simulink model "p1_digital_twin_R2023a"  (R2023a)
settings: Solver=FixedStepDiscrete  StartTime=0.0  StopTime=10  FixedStep=Ts  RelTol=1e-3  EnableMultiTasking=on
values from neighbouring files (symbols this model uses):
  ack = 1    [SteeringController.m]
  cpr_handwheel = 500*4    (= 2000)    [p1_params_new.m]
  cpr_steering = 1000*4    (= 4000)    [p1_params_new.m]
  hal_filter_den = [1 1*(2*pi*Ts)-1]    [SteeringController.m]    (also in p1_params_new.m = DEN_cellarray{1})
  hal_filter_num = [1*(2*pi*Ts)]    [SteeringController.m]    (also in p1_params_new.m = NUM_cellarray{1})
  n_drive = 5.6    [p1_params_new.m]
  n_handwheel = 50    [p1_params_new.m]
  n_steering = 160    [p1_params_new.m]
  sr = 7.5    [SteeringController.m]
  steering_limit = 35    [SteeringController.m]
  Ts = 0.001    [p1_params_new.m]
  wc = 10    [SteeringController.m]    (also in p1_params_new.m = p1params.input.VAccelFc*(2*Ts))
undefined symbols (not defined in the file or in its folder): DiscIntNeverNeededParam, p1params, param
libraries: simulink x7
(part 3 of 4)

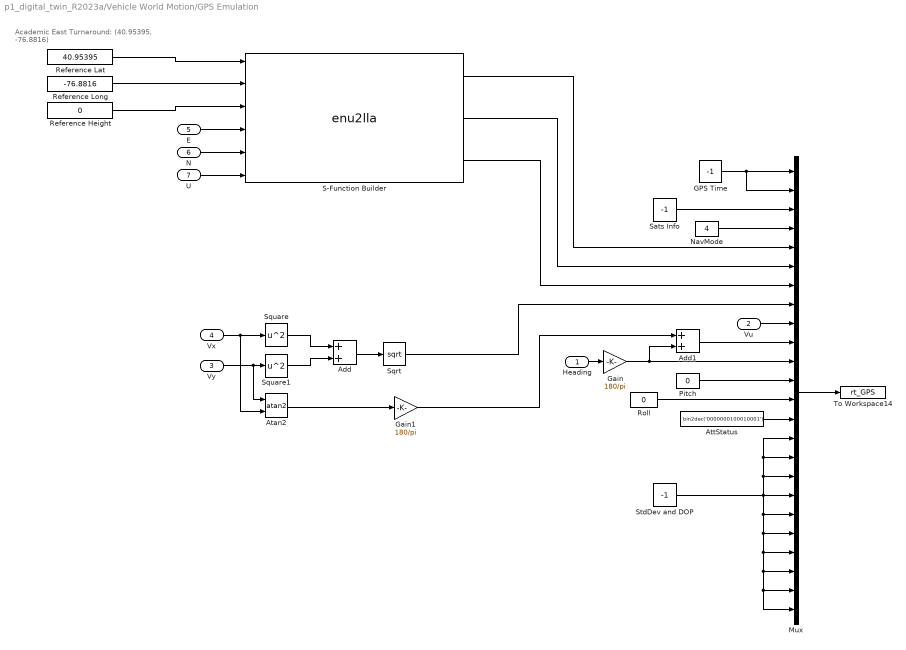
== system p1_digital_twin_R2023a/Vehicle World Motion/GPS Emulation ==
  note: Academic East Turnaround:
      | (40.95395, -76.8816)
  Heading : Inport
  Vu : Inport  Port=2
  Vy : Inport  Port=3
  Vx : Inport  Port=4
  E : Inport  Port=5
  N : Inport  Port=6
  U : Inport  Port=7
  Add : Sum
  Add1 : Sum
  Atan2 : Trigonometry  Operator=atan2
  AttStatus : Constant  Value=bin2dec('0000000100010001')  OutDataTypeStr=double
  GPS Time : Constant  Value=-1
  Gain : Gain  Gain=180/pi
  Gain1 : Gain  Gain=180/pi
  Mux : Mux  Inputs=24
  NavMode : Constant  Value=4
  Pitch : Constant  Value=0
  Reference Height : Constant  Value=0
  Reference Lat : Constant  Value=40.95395
  Reference Long : Constant  Value=-76.8816
  Roll : Constant  Value=0
  S-Function Builder : S-Function  FunctionName=enu2lla  SFunctionModules=enu2lla_wrapper.c  SFunctionDeploymentMode=off  EnableBusSupport=off  mask(S-Function Builder){}
      mask help: Simulink:masks:SFunctionBuilder_MD
      mask init: same as p1_digital_twin_R2023a/Actuator Dynamics/Steering System Emulation/S-Function Builder1
      settings: CopyFcn=set_param(gcbh,'LinkStatus','none')  OpenFcn=sfunctionwizard(gcbh)
      mask Display:
      | plot(val(:,1),val(:,2))
      | disp(sys)
      | port_label('input',1,'u0')
      | port_label('input',2,'u1')
      | port_label('input',3,'u2')
      | port_label('input',4,'u3')
      | port_label('input',5,'u4')
      | port_label('input',6,'u5')
      | port_label('output',1,'y0')
      | port_label('output',2,'y1')
      | port_label('output',3,'y2')
  Sats Info : Constant  Value=-1
  Sqrt : Sqrt
  Square : Math  Operator=square
  Square1 : Math  Operator=square
  StdDev and DOP : Constant  Value=-1
  To Workspace14 : ToWorkspace  VariableName=rt_GPS  SampleTime=-1
  wires:
  Add/1 -> Sqrt/1
  Vy/1 -> Atan2/1, Square1/1
  Vx/1 -> Atan2/2, Square/1
  Square/1 -> Add/1
  Square1/1 -> Add/2
  GPS Time/1 -> Mux/1, Mux/2
  NavMode/1 -> Mux/4
  S-Function Builder/1 -> Mux/5
  Sqrt/1 -> Mux/8
  Vu/1 -> Mux/9
  S-Function Builder/2 -> Mux/6
  S-Function Builder/3 -> Mux/7
  Pitch/1 -> Mux/12
  AttStatus/1 -> Mux/14
  Heading/1 -> Gain/1
  StdDev and DOP/1 -> Mux/18, Mux/17, Mux/16, Mux/15, Mux/19, Mux/20, Mux/21, Mux/22, Mux/23, Mux/24
  Sats Info/1 -> Mux/3
  Mux/1 -> To Workspace14/1
  Roll/1 -> Mux/13
  Gain/1 -> Add1/2, Mux/11
  Atan2/1 -> Gain1/1
  Add1/1 -> Mux/10
  Gain1/1 -> Add1/1
  Reference Lat/1 -> S-Function Builder/1
  Reference Long/1 -> S-Function Builder/2
  Reference Height/1 -> S-Function Builder/3
  E/1 -> S-Function Builder/4
  U/1 -> S-Function Builder/6
  N/1 -> S-Function Builder/5

== system p1_digital_twin_R2023a/Vehicle World Motion/IMU Emulation1 ==
  note: Filtering Operations from IMU?
  note: Break into bytes
  Roll Rate : Inport
  Pitch Rate : Inport  Port=2
  Yaw Rate : Inport  Port=3
  Ax : Inport  Port=4
  Ay : Inport  Port=5
  Az : Inport  Port=6
  Accel unscaling : Gain  Gain=32768/(2*9.81)
  Accel unscaling1 : Gain  Gain=32768/(2*9.81)
  Accel unscaling2 : Gain  Gain=32768/(2*9.81)
  Data Type Conversion{,1..5} (6 alike) : DataTypeConversion  OutDataTypeStr=int16  SaturateOnIntegerOverflow=off  RndMeth=Floor
  Gyro unscaling : Gain  Gain=32768/(500*pi/180)
  Gyro unscaling1 : Gain  Gain=32768/500
  Gyro unscaling2 : Gain  Gain=32768/500
  Mux : Mux  Inputs=12
  S-Function Builder : S-Function  FunctionName=int16ToBytes  SFunctionModules=int16ToBytes_wrapper.c  SFunctionDeploymentMode=off  EnableBusSupport=off  mask(S-Function Builder){}
      mask help: Simulink:masks:SFunctionBuilder_MD
      mask init: same as p1_digital_twin_R2023a/Actuator Dynamics/Steering System Emulation/S-Function Builder1
      settings: CopyFcn=set_param(gcbh,'LinkStatus','none')  OpenFcn=sfunctionwizard(gcbh)
      mask Display:
      | plot(val(:,1),val(:,2))
      | disp(sys)
      | port_label('input',1,'u0')
      | port_label('output',1,'y0')
  S-Function Builder1 : S-Function  FunctionName=int16ToBytes  SFunctionModules=int16ToBytes_wrapper.c  SFunctionDeploymentMode=off  EnableBusSupport=off  mask(S-Function Builder){}
      mask help: Simulink:masks:SFunctionBuilder_MD
      mask init: same as p1_digital_twin_R2023a/Actuator Dynamics/Steering System Emulation/S-Function Builder1
      settings: CopyFcn=set_param(gcbh,'LinkStatus','none')  OpenFcn=sfunctionwizard(gcbh)
      mask Display:
      | plot(val(:,1),val(:,2))
      | disp(sys)
      | port_label('input',1,'u0')
      | port_label('output',1,'y0')
  S-Function Builder2 : S-Function  FunctionName=int16ToBytes  SFunctionModules=int16ToBytes_wrapper.c  SFunctionDeploymentMode=off  EnableBusSupport=off  mask(S-Function Builder){}
      mask help: Simulink:masks:SFunctionBuilder_MD
      mask init: same as p1_digital_twin_R2023a/Actuator Dynamics/Steering System Emulation/S-Function Builder1
      settings: CopyFcn=set_param(gcbh,'LinkStatus','none')  OpenFcn=sfunctionwizard(gcbh)
      mask Display:
      | plot(val(:,1),val(:,2))
      | disp(sys)
      | port_label('input',1,'u0')
      | port_label('output',1,'y0')
      | port_label('output',2,'y1')
  S-Function Builder3 : S-Function  FunctionName=int16ToBytes  SFunctionModules=int16ToBytes_wrapper.c  SFunctionDeploymentMode=off  EnableBusSupport=off  mask(S-Function Builder){}
      mask help: Simulink:masks:SFunctionBuilder_MD
      mask init: same as p1_digital_twin_R2023a/Actuator Dynamics/Steering System Emulation/S-Function Builder1
      settings: CopyFcn=set_param(gcbh,'LinkStatus','none')  OpenFcn=sfunctionwizard(gcbh)
      mask Display:
      | plot(val(:,1),val(:,2))
      | disp(sys)
      | port_label('input',1,'u0')
      | port_label('output',1,'y0')
  S-Function Builder4 : S-Function  FunctionName=int16ToBytes  SFunctionModules=int16ToBytes_wrapper.c  SFunctionDeploymentMode=off  EnableBusSupport=off  mask(S-Function Builder){}
      mask help: Simulink:masks:SFunctionBuilder_MD
      mask init: same as p1_digital_twin_R2023a/Actuator Dynamics/Steering System Emulation/S-Function Builder1
      settings: CopyFcn=set_param(gcbh,'LinkStatus','none')  OpenFcn=sfunctionwizard(gcbh)
      mask Display:
      | plot(val(:,1),val(:,2))
      | disp(sys)
      | port_label('input',1,'u0')
      | port_label('output',1,'y0')
  S-Function Builder5 : S-Function  FunctionName=int16ToBytes  SFunctionModules=int16ToBytes_wrapper.c  SFunctionDeploymentMode=off  EnableBusSupport=off  mask(S-Function Builder){}
      mask help: Simulink:masks:SFunctionBuilder_MD
      mask init: same as p1_digital_twin_R2023a/Actuator Dynamics/Steering System Emulation/S-Function Builder1
      settings: CopyFcn=set_param(gcbh,'LinkStatus','none')  OpenFcn=sfunctionwizard(gcbh)
      mask Display:
      | plot(val(:,1),val(:,2))
      | disp(sys)
      | port_label('input',1,'u0')
      | port_label('output',1,'y0')
  To Workspace16 : ToWorkspace  VariableName=rt_IMU  SampleTime=-1
      settings: Save2DSignal=2-D array (concatenate along first dimension)
  wires:
  Mux/1 -> To Workspace16/1
  Accel unscaling/1 -> Data Type Conversion3/1
  Accel unscaling1/1 -> Data Type Conversion4/1
  Accel unscaling2/1 -> Data Type Conversion5/1
  Gyro unscaling2/1 -> Data Type Conversion2/1
  Pitch Rate/1 -> Gyro unscaling1/1
  Yaw Rate/1 -> Gyro unscaling/1
  Gyro unscaling1/1 -> Data Type Conversion1/1
  Gyro unscaling/1 -> Data Type Conversion/1
  Roll Rate/1 -> Gyro unscaling2/1
  Az/1 -> Accel unscaling2/1
  Ay/1 -> Accel unscaling1/1
  Ax/1 -> Accel unscaling/1
  Data Type Conversion/1 -> S-Function Builder/1
  Data Type Conversion2/1 -> S-Function Builder2/1
  Data Type Conversion1/1 -> S-Function Builder1/1
  Data Type Conversion3/1 -> S-Function Builder3/1
  Data Type Conversion4/1 -> S-Function Builder4/1
  Data Type Conversion5/1 -> S-Function Builder5/1
  S-Function Builder5/1 -> Mux/11, Mux/12
  S-Function Builder2/1 -> Mux/1, Mux/2
  S-Function Builder1/1 -> Mux/3, Mux/4
  S-Function Builder/1 -> Mux/5, Mux/6
  S-Function Builder3/1 -> Mux/7, Mux/8
  S-Function Builder4/1 -> Mux/9, Mux/10

== system p1_digital_twin_R2023a/Actuator Dynamics/Drivetrain Emulation/Accurate Feedback L ==
  Actual Torque : Inport
  Actual Voltage : Inport  Port=2
  Actual Current : Inport  Port=3
  Actual Speed : Inport  Port=4
  Bias1 : Bias  Bias=3212.8  SaturateOnIntegerOverflow=off
  Bias2 : Bias  Bias=3212.8  SaturateOnIntegerOverflow=off
  Bias3 : Bias  Bias=16064  SaturateOnIntegerOverflow=off
  Data Type Conversion{1..3,5} (4 alike) : DataTypeConversion  OutDataTypeStr=uint16  SaturateOnIntegerOverflow=off  RndMeth=Floor
  Mux{,1,3..4} (4 alike) : Mux  Inputs=2
  Mux2 : Mux
  S-Function Builder : S-Function  FunctionName=uint16ToBytes  SFunctionModules=uint16ToBytes_wrapper.c  SFunctionDeploymentMode=off  EnableBusSupport=off  mask(S-Function Builder){}
      mask help: Simulink:masks:SFunctionBuilder_MD
      mask init: same as p1_digital_twin_R2023a/Actuator Dynamics/Steering System Emulation/S-Function Builder1
      settings: CopyFcn=set_param(gcbh,'LinkStatus','none')  OpenFcn=sfunctionwizard(gcbh)
      mask Display:
      | plot(val(:,1),val(:,2))
      | disp(sys)
      | port_label('input',1,'u0')
      | port_label('output',1,'y0')
      | port_label('output',2,'y1')
  S-Function Builder1 : S-Function  FunctionName=uint16ToBytes  SFunctionModules=uint16ToBytes_wrapper.c  SFunctionDeploymentMode=off  EnableBusSupport=off  mask(S-Function Builder){}
      mask help: Simulink:masks:SFunctionBuilder_MD
      mask init: same as p1_digital_twin_R2023a/Actuator Dynamics/Steering System Emulation/S-Function Builder1
      settings: CopyFcn=set_param(gcbh,'LinkStatus','none')  OpenFcn=sfunctionwizard(gcbh)
      mask Display:
      | plot(val(:,1),val(:,2))
      | disp(sys)
      | port_label('input',1,'u0')
      | port_label('output',1,'y0')
      | port_label('output',2,'y1')
  S-Function Builder2 : S-Function  FunctionName=uint16ToBytes  SFunctionModules=uint16ToBytes_wrapper.c  SFunctionDeploymentMode=off  EnableBusSupport=off  mask(S-Function Builder){}
      mask help: Simulink:masks:SFunctionBuilder_MD
      mask init: same as p1_digital_twin_R2023a/Actuator Dynamics/Steering System Emulation/S-Function Builder1
      settings: CopyFcn=set_param(gcbh,'LinkStatus','none')  OpenFcn=sfunctionwizard(gcbh)
      mask Display:
      | plot(val(:,1),val(:,2))
      | disp(sys)
      | port_label('input',1,'u0')
      | port_label('output',1,'y0')
      | port_label('output',2,'y1')
  S-Function Builder3 : S-Function  FunctionName=uint16ToBytes  SFunctionModules=uint16ToBytes_wrapper.c  SFunctionDeploymentMode=off  EnableBusSupport=off  mask(S-Function Builder){}
      mask help: Simulink:masks:SFunctionBuilder_MD
      mask init: same as p1_digital_twin_R2023a/Actuator Dynamics/Steering System Emulation/S-Function Builder1
      settings: CopyFcn=set_param(gcbh,'LinkStatus','none')  OpenFcn=sfunctionwizard(gcbh)
      mask Display:
      | plot(val(:,1),val(:,2))
      | disp(sys)
      | port_label('input',1,'u0')
      | port_label('output',1,'y0')
      | port_label('output',2,'y1')
  Speed scaling1 : Gain  Gain=1/.1
  Speed scaling2 : Gain  Gain=1/.1
  Speed scaling3 : Gain  Gain=1/.5
  Torque offset : Bias  Bias=+3212.8  SaturateOnIntegerOverflow=off
  Torque scaling : Gain  Gain=1/.1
  Out2 : Outport
  wires:
  Mux2/1 -> Out2/1
  Actual Torque/1 -> Torque offset/1
  Torque scaling/1 -> Data Type Conversion5/1
  Data Type Conversion5/1 -> S-Function Builder3/1
  S-Function Builder3/2 -> Mux/2
  S-Function Builder3/1 -> Mux/1
  Mux/1 -> Mux2/1
  S-Function Builder2/1 -> Mux1/1
  Speed scaling1/1 -> Data Type Conversion1/1
  Actual Voltage/1 -> Bias1/1
  S-Function Builder2/2 -> Mux1/2
  Mux1/1 -> Mux2/2
  Data Type Conversion1/1 -> S-Function Builder2/1
  S-Function Builder1/2 -> Mux3/2
  Speed scaling2/1 -> Data Type Conversion2/1
  Data Type Conversion2/1 -> S-Function Builder1/1
  Actual Current/1 -> Bias2/1
  S-Function Builder1/1 -> Mux3/1
  Mux3/1 -> Mux2/3
  Torque offset/1 -> Torque scaling/1
  Bias1/1 -> Speed scaling1/1
  Bias2/1 -> Speed scaling2/1
  S-Function Builder/2 -> Mux4/2
  Mux4/1 -> Mux2/4
  Speed scaling3/1 -> Data Type Conversion3/1
  Data Type Conversion3/1 -> S-Function Builder/1
  Bias3/1 -> Speed scaling3/1
  Actual Speed/1 -> Bias3/1
  S-Function Builder/1 -> Mux4/1

== system p1_digital_twin_R2023a/Actuator Dynamics/Drivetrain Emulation/Accurate Feedback R ==
  Actual Torque : Inport
  Actual Voltage : Inport  Port=2
  Actual Current : Inport  Port=3
  Actual Speed : Inport  Port=4
  Bias1 : Bias  Bias=3212.8  SaturateOnIntegerOverflow=off
  Bias2 : Bias  Bias=3212.8  SaturateOnIntegerOverflow=off
  Bias3 : Bias  Bias=16064  SaturateOnIntegerOverflow=off
  Data Type Conversion{1..3,5} (4 alike) : DataTypeConversion  OutDataTypeStr=uint16  SaturateOnIntegerOverflow=off  RndMeth=Floor
  Mux{,1,3..4} (4 alike) : Mux  Inputs=2
  Mux2 : Mux
  S-Function Builder : S-Function  FunctionName=uint16ToBytes  SFunctionModules=uint16ToBytes_wrapper.c  SFunctionDeploymentMode=off  EnableBusSupport=off  mask(S-Function Builder){}
      mask help: Simulink:masks:SFunctionBuilder_MD
      mask init: same as p1_digital_twin_R2023a/Actuator Dynamics/Steering System Emulation/S-Function Builder1
      settings: CopyFcn=set_param(gcbh,'LinkStatus','none')  OpenFcn=sfunctionwizard(gcbh)
      mask Display:
      | plot(val(:,1),val(:,2))
      | disp(sys)
      | port_label('input',1,'u0')
      | port_label('output',1,'y0')
      | port_label('output',2,'y1')
  S-Function Builder1 : S-Function  FunctionName=uint16ToBytes  SFunctionModules=uint16ToBytes_wrapper.c  SFunctionDeploymentMode=off  EnableBusSupport=off  mask(S-Function Builder){}
      mask help: Simulink:masks:SFunctionBuilder_MD
      mask init: same as p1_digital_twin_R2023a/Actuator Dynamics/Steering System Emulation/S-Function Builder1
      settings: CopyFcn=set_param(gcbh,'LinkStatus','none')  OpenFcn=sfunctionwizard(gcbh)
      mask Display:
      | plot(val(:,1),val(:,2))
      | disp(sys)
      | port_label('input',1,'u0')
      | port_label('output',1,'y0')
      | port_label('output',2,'y1')
  S-Function Builder2 : S-Function  FunctionName=uint16ToBytes  SFunctionModules=uint16ToBytes_wrapper.c  SFunctionDeploymentMode=off  EnableBusSupport=off  mask(S-Function Builder){}
      mask help: Simulink:masks:SFunctionBuilder_MD
      mask init: same as p1_digital_twin_R2023a/Actuator Dynamics/Steering System Emulation/S-Function Builder1
      settings: CopyFcn=set_param(gcbh,'LinkStatus','none')  OpenFcn=sfunctionwizard(gcbh)
      mask Display:
      | plot(val(:,1),val(:,2))
      | disp(sys)
      | port_label('input',1,'u0')
      | port_label('output',1,'y0')
      | port_label('output',2,'y1')
  S-Function Builder3 : S-Function  FunctionName=uint16ToBytes  SFunctionModules=uint16ToBytes_wrapper.c  SFunctionDeploymentMode=off  EnableBusSupport=off  mask(S-Function Builder){}
      mask help: Simulink:masks:SFunctionBuilder_MD
      mask init: same as p1_digital_twin_R2023a/Actuator Dynamics/Steering System Emulation/S-Function Builder1
      settings: CopyFcn=set_param(gcbh,'LinkStatus','none')  OpenFcn=sfunctionwizard(gcbh)
      mask Display:
      | plot(val(:,1),val(:,2))
      | disp(sys)
      | port_label('input',1,'u0')
      | port_label('output',1,'y0')
      | port_label('output',2,'y1')
  Speed scaling1 : Gain  Gain=1/.1
  Speed scaling2 : Gain  Gain=1/.1
  Speed scaling3 : Gain  Gain=1/.5
  Torque offset : Bias  Bias=+3212.8  SaturateOnIntegerOverflow=off
  Torque scaling : Gain  Gain=1/.1
  Out2 : Outport
  wires:
  Mux2/1 -> Out2/1
  Actual Torque/1 -> Torque offset/1
  Torque scaling/1 -> Data Type Conversion5/1
  Data Type Conversion5/1 -> S-Function Builder3/1
  S-Function Builder3/2 -> Mux/2
  S-Function Builder3/1 -> Mux/1
  Mux/1 -> Mux2/1
  S-Function Builder2/1 -> Mux1/1
  Speed scaling1/1 -> Data Type Conversion1/1
  Actual Voltage/1 -> Bias1/1
  S-Function Builder2/2 -> Mux1/2
  Mux1/1 -> Mux2/2
  Data Type Conversion1/1 -> S-Function Builder2/1
  S-Function Builder1/2 -> Mux3/2
  Speed scaling2/1 -> Data Type Conversion2/1
  Data Type Conversion2/1 -> S-Function Builder1/1
  Actual Current/1 -> Bias2/1
  S-Function Builder1/1 -> Mux3/1
  Mux3/1 -> Mux2/3
  Torque offset/1 -> Torque scaling/1
  Bias1/1 -> Speed scaling1/1
  Bias2/1 -> Speed scaling2/1
  S-Function Builder/2 -> Mux4/2
  Mux4/1 -> Mux2/4
  Speed scaling3/1 -> Data Type Conversion3/1
  Data Type Conversion3/1 -> S-Function Builder/1
  Bias3/1 -> Speed scaling3/1
  Actual Speed/1 -> Bias3/1
  S-Function Builder/1 -> Mux4/1

== system p1_digital_twin_R2023a/Actuator Dynamics/Drivetrain Emulation/Universal Command L ==
  Torque Request : Inport
  Fwd Speed Lim : Inport  Port=2
  Rev Speed Lim : Inport  Port=3
  Bias1 : Bias  Bias=16064  SaturateOnIntegerOverflow=off
  Bias2 : Bias  Bias=16064  SaturateOnIntegerOverflow=off
  Control Mode : Constant  Value=hex2dec('01')  OutDataTypeStr=uint8  SampleTime=-1
  Control Params : Constant  Value=bin2dec('00011000')  OutDataTypeStr=uint8  SampleTime=-1
  Data Type Conversion1 : DataTypeConversion  OutDataTypeStr=uint16  RndMeth=Floor
  Data Type Conversion2 : DataTypeConversion  OutDataTypeStr=uint16  SaturateOnIntegerOverflow=off  RndMeth=Floor
  Data Type Conversion5 : DataTypeConversion  OutDataTypeStr=uint16  SaturateOnIntegerOverflow=off  RndMeth=Floor
  Mux : Mux  Inputs=2
  Mux1 : Mux  Inputs=2
  Mux2 : Mux  Inputs=5
  Mux3 : Mux  Inputs=2
  S-Function Builder1 : S-Function  FunctionName=uint16ToBytes  SFunctionModules=uint16ToBytes_wrapper.c  SFunctionDeploymentMode=off  EnableBusSupport=off  mask(S-Function Builder){}
      mask help: Simulink:masks:SFunctionBuilder_MD
      mask init: same as p1_digital_twin_R2023a/Actuator Dynamics/Steering System Emulation/S-Function Builder1
      settings: CopyFcn=set_param(gcbh,'LinkStatus','none')  OpenFcn=sfunctionwizard(gcbh)
      mask Display:
      | plot(val(:,1),val(:,2))
      | disp(sys)
      | port_label('input',1,'u0')
      | port_label('output',1,'y0')
      | port_label('output',2,'y1')
  S-Function Builder2 : S-Function  FunctionName=uint16ToBytes  SFunctionModules=uint16ToBytes_wrapper.c  SFunctionDeploymentMode=off  EnableBusSupport=off  mask(S-Function Builder){}
      mask help: Simulink:masks:SFunctionBuilder_MD
      mask init: same as p1_digital_twin_R2023a/Actuator Dynamics/Steering System Emulation/S-Function Builder1
      settings: CopyFcn=set_param(gcbh,'LinkStatus','none')  OpenFcn=sfunctionwizard(gcbh)
      mask Display:
      | plot(val(:,1),val(:,2))
      | disp(sys)
      | port_label('input',1,'u0')
      | port_label('output',1,'y0')
      | port_label('output',2,'y1')
  S-Function Builder3 : S-Function  FunctionName=uint16ToBytes  SFunctionModules=uint16ToBytes_wrapper.c  SFunctionDeploymentMode=off  EnableBusSupport=off  mask(S-Function Builder){}
      mask help: Simulink:masks:SFunctionBuilder_MD
      mask init: same as p1_digital_twin_R2023a/Actuator Dynamics/Steering System Emulation/S-Function Builder1
      settings: CopyFcn=set_param(gcbh,'LinkStatus','none')  OpenFcn=sfunctionwizard(gcbh)
      mask Display:
      | plot(val(:,1),val(:,2))
      | disp(sys)
      | port_label('input',1,'u0')
      | port_label('output',1,'y0')
      | port_label('output',2,'y1')
  Speed scaling1 : Gain  Gain=1/.5
  Speed scaling2 : Gain  Gain=1/.5
  Torque offset : Bias  Bias=+3212.8  SaturateOnIntegerOverflow=off
  Torque scaling : Gain  Gain=1/.1
  Out2 : Outport
  wires:
  Mux2/1 -> Out2/1
  Torque Request/1 -> Torque offset/1
  Control Mode/1 -> Mux2/1
  Control Params/1 -> Mux2/2
  Torque scaling/1 -> Data Type Conversion5/1
  Data Type Conversion5/1 -> S-Function Builder3/1
  S-Function Builder3/2 -> Mux/2
  S-Function Builder3/1 -> Mux/1
  Mux/1 -> Mux2/3
  S-Function Builder2/1 -> Mux1/1
  Speed scaling1/1 -> Data Type Conversion1/1
  Fwd Speed Lim/1 -> Bias1/1
  S-Function Builder2/2 -> Mux1/2
  Mux1/1 -> Mux2/4
  Data Type Conversion1/1 -> S-Function Builder2/1
  S-Function Builder1/2 -> Mux3/2
  Speed scaling2/1 -> Data Type Conversion2/1
  Data Type Conversion2/1 -> S-Function Builder1/1
  Rev Speed Lim/1 -> Bias2/1
  S-Function Builder1/1 -> Mux3/1
  Mux3/1 -> Mux2/5
  Torque offset/1 -> Torque scaling/1
  Bias1/1 -> Speed scaling1/1
  Bias2/1 -> Speed scaling2/1

== system p1_digital_twin_R2023a/Actuator Dynamics/Drivetrain Emulation/Universal Command R ==
  Torque Request : Inport
  Fwd Speed Lim : Inport  Port=2
  Rev Speed Lim : Inport  Port=3
  Bias1 : Bias  Bias=16064  SaturateOnIntegerOverflow=off
  Bias2 : Bias  Bias=16064  SaturateOnIntegerOverflow=off
  Control Mode : Constant  Value=hex2dec('01')  OutDataTypeStr=uint8  SampleTime=-1
  Control Params : Constant  Value=bin2dec('00011000')  OutDataTypeStr=uint8  SampleTime=-1
  Data Type Conversion1 : DataTypeConversion  OutDataTypeStr=uint16  SaturateOnIntegerOverflow=off  RndMeth=Floor
  Data Type Conversion2 : DataTypeConversion  OutDataTypeStr=uint16  SaturateOnIntegerOverflow=off  RndMeth=Floor
  Data Type Conversion5 : DataTypeConversion  OutDataTypeStr=uint16  SaturateOnIntegerOverflow=off  RndMeth=Floor
  Mux : Mux  Inputs=2
  Mux1 : Mux  Inputs=2
  Mux2 : Mux  Inputs=5
  Mux3 : Mux  Inputs=2
  S-Function Builder1 : S-Function  FunctionName=uint16ToBytes  SFunctionModules=uint16ToBytes_wrapper.c  SFunctionDeploymentMode=off  EnableBusSupport=off  mask(S-Function Builder){}
      mask help: Simulink:masks:SFunctionBuilder_MD
      mask init: same as p1_digital_twin_R2023a/Actuator Dynamics/Steering System Emulation/S-Function Builder1
      settings: CopyFcn=set_param(gcbh,'LinkStatus','none')  OpenFcn=sfunctionwizard(gcbh)
      mask Display:
      | plot(val(:,1),val(:,2))
      | disp(sys)
      | port_label('input',1,'u0')
      | port_label('output',1,'y0')
      | port_label('output',2,'y1')
  S-Function Builder2 : S-Function  FunctionName=uint16ToBytes  SFunctionModules=uint16ToBytes_wrapper.c  SFunctionDeploymentMode=off  EnableBusSupport=off  mask(S-Function Builder){}
      mask help: Simulink:masks:SFunctionBuilder_MD
      mask init: same as p1_digital_twin_R2023a/Actuator Dynamics/Steering System Emulation/S-Function Builder1
      settings: CopyFcn=set_param(gcbh,'LinkStatus','none')  OpenFcn=sfunctionwizard(gcbh)
      mask Display:
      | plot(val(:,1),val(:,2))
      | disp(sys)
      | port_label('input',1,'u0')
      | port_label('output',1,'y0')
      | port_label('output',2,'y1')
  S-Function Builder3 : S-Function  FunctionName=uint16ToBytes  SFunctionModules=uint16ToBytes_wrapper.c  SFunctionDeploymentMode=off  EnableBusSupport=off  mask(S-Function Builder){}
      mask help: Simulink:masks:SFunctionBuilder_MD
      mask init: same as p1_digital_twin_R2023a/Actuator Dynamics/Steering System Emulation/S-Function Builder1
      settings: CopyFcn=set_param(gcbh,'LinkStatus','none')  OpenFcn=sfunctionwizard(gcbh)
      mask Display:
      | plot(val(:,1),val(:,2))
      | disp(sys)
      | port_label('input',1,'u0')
      | port_label('output',1,'y0')
      | port_label('output',2,'y1')
  Speed scaling1 : Gain  Gain=1/.5
  Speed scaling2 : Gain  Gain=1/.5
  Torque offset : Bias  Bias=+3212.8  SaturateOnIntegerOverflow=off
  Torque scaling : Gain  Gain=1/.1
  Out2 : Outport
  wires:
  Mux2/1 -> Out2/1
  Torque Request/1 -> Torque offset/1
  Control Mode/1 -> Mux2/1
  Control Params/1 -> Mux2/2
  Torque scaling/1 -> Data Type Conversion5/1
  Data Type Conversion5/1 -> S-Function Builder3/1
  S-Function Builder3/2 -> Mux/2
  S-Function Builder3/1 -> Mux/1
  Mux/1 -> Mux2/3
  S-Function Builder2/1 -> Mux1/1
  Speed scaling1/1 -> Data Type Conversion1/1
  Fwd Speed Lim/1 -> Bias1/1
  S-Function Builder2/2 -> Mux1/2
  Mux1/1 -> Mux2/4
  Data Type Conversion1/1 -> S-Function Builder2/1
  S-Function Builder1/2 -> Mux3/2
  Speed scaling2/1 -> Data Type Conversion2/1
  Data Type Conversion2/1 -> S-Function Builder1/1
  Rev Speed Lim/1 -> Bias2/1
  S-Function Builder1/1 -> Mux3/1
  Mux3/1 -> Mux2/5
  Torque offset/1 -> Torque scaling/1
  Bias1/1 -> Speed scaling1/1
  Bias2/1 -> Speed scaling2/1

== system p1_digital_twin_R2023a/Actuator Dynamics/Left Steering Model/PID Current ==
  In2 : Inport
  In1 : Inport  Port=2
  Add10 : Sum  Inputs=+++
  Discrete Derivative : simulink/Discrete/Discrete Derivative  gainval=1  ICPrevScaledInput=0.0  OutMin=[]  OutMax=[]  OutDataType=fixdt(1, 16)  OutScaling=2^-10  DoSatur=off
  Discrete-Time Integrator : DiscreteIntegrator  gainval=1  SampleTime=-1  ICPrevOutput=DiscIntNeverNeededParam  ICPrevScaledInput=DiscIntNeverNeededParam
  Kd : Constant  Value=40
  Ki : Constant  Value=2500
  Kp : Constant  Value=3000
  Product : Product
  Product20 : Product
  Product21 : Product
  Subtract8 : Sum  Inputs=+-
  Out1 : Outport
  wires:
  In2/1 -> Subtract8/1
  Subtract8/1 -> Discrete Derivative/1, Discrete-Time Integrator/1, Product20/2
  Ki/1 -> Product21/1
  Kp/1 -> Product20/1
  Discrete-Time Integrator/1 -> Product21/2
  Product21/1 -> Add10/2
  Product20/1 -> Add10/1
  Add10/1 -> Out1/1
  In1/1 -> Subtract8/2
  Discrete Derivative/1 -> Product/1
  Kd/1 -> Product/2
  Product/1 -> Add10/3

== system p1_digital_twin_R2023a/Actuator Dynamics/Right Steering Model/PID Current ==
  In2 : Inport
  In1 : Inport  Port=2
  Add10 : Sum  Inputs=+++
  Discrete Derivative : simulink/Discrete/Discrete Derivative  gainval=1.0  ICPrevScaledInput=0.0  OutMin=[]  OutMax=[]  OutDataType=fixdt(1, 16)  OutScaling=2^-10  DoSatur=off
  Discrete-Time Integrator : DiscreteIntegrator  gainval=1  SampleTime=-1  ICPrevOutput=DiscIntNeverNeededParam  ICPrevScaledInput=DiscIntNeverNeededParam
  Kd : Constant  Value=100
  Ki : Constant  Value=100
  Kp : Constant  Value=5000
  Product : Product
  Product20 : Product
  Product21 : Product
  Subtract8 : Sum  Inputs=+-
  Out1 : Outport
  wires:
  In2/1 -> Subtract8/1
  Subtract8/1 -> Discrete Derivative/1, Discrete-Time Integrator/1, Product20/2
  Ki/1 -> Product21/1
  Kp/1 -> Product20/1
  Discrete-Time Integrator/1 -> Product21/2
  Product21/1 -> Add10/2
  Product20/1 -> Add10/1
  Add10/1 -> Out1/1
  In1/1 -> Subtract8/2
  Discrete Derivative/1 -> Product/1
  Kd/1 -> Product/2
  Product/1 -> Add10/3

== system p1_digital_twin_R2023a/Driver and Controller Input/Steering Controller/Ackermann Correction ==
  Ackermann Angle : Inport
  left ackermann ideal correction angle : Fcn  Expr=u/(1-u*ack*param.d/2/(param.a+param.b))
  right ackermann ideal correction angle : Fcn  Expr=u/(1+u*ack*param.d/2/(param.a+param.b))
  L Steer Angle : Outport
  R Steer Angle : Outport  Port=2
  wires:
  Ackermann Angle/1 -> right ackermann ideal correction angle/1, left ackermann ideal correction angle/1
  right ackermann ideal correction angle/1 -> R Steer Angle/1
  left ackermann ideal correction angle/1 -> L Steer Angle/1

== system p1_digital_twin_R2023a/Driver and Controller Input/Steering Controller/HAL-9000 ==
  Trigger : Inport
  Amplitude : Constant  Value=amplitude*sr*pi/180
  Chirp Signal : Subsystem  mask(chirp){f1=startfreq, T=duration, f2=endfreq, VectorParams1D=on}
      mask prompts: f1 "Initial frequency (Hz):"; T "Target time (secs):"; f2 "Frequency at target time (Hz):"; VectorParams1D "Interpret vectors parameters as 1-D"
      mask help: Output a linear chirp signal (sine wave whose frequency varies linearly with time).
      mask init:
      | blkName = gcb;
      | t=[0:.1:5];
      | set_param([blkName '/targetTime'], 'VectorParams1D', VectorParams1D);
      | set_param([blkName '/initialFreq'], 'VectorParams1D', VectorParams1D);
      | set_param([blkName '/deltaFreq'], 'VectorParams1D', VectorParams1D);
      mask Help: The chirp signal has linearly increasing frequency with time.  This block can be used for spectral analysis of nonlinear systems.
      mask Display: plot(t,sin(t.*t))
  Constant : Constant
  Constant1 : Constant  Value=0
  Delay : Constant  Value=delay
  Digital Clock : DigitalClock  SampleTime=Ts
  Double chirp : Subsystem
  Double-step : Subsystem
      mask Display: plot([0 1 1 2 2 3 3 4 4 5],[0 0 1 1 0 0 -1 -1 0 0])
  Enable : Constant  Value=enabled
  Latch : Subsystem  TreatAsAtomicUnit=on
  Maneuver : Constant  Value=maneuver
  Multiport Switch : MultiPortSwitch  Inputs=5  SaturateOnIntegerOverflow=off  InputSameDT=off
  Product : Product  Inputs=3  SaturateOnIntegerOverflow=on  OutDataTypeStr=Inherit: Same as first input
  Product1 : Product  SaturateOnIntegerOverflow=on  OutDataTypeStr=Inherit: Same as first input
  Ramp : Subsystem
      mask Display: plot([0 3 7 10],[1 1 8 8])
  Step : Subsystem
      mask Display: plot([0 5 5 10],[1 1 8 8])
  Sum : Sum  Inputs=|++
  Switch : Switch  Criteria=u2 ~= 0  SaturateOnIntegerOverflow=off  InputSameDT=off
  Offset : Outport
  wires:
  Double chirp/1(Out1) -> Multiport Switch/6
  Double-step/1(Out) -> Multiport Switch/5
  Enable/1 -> Product1/2
  Trigger/1 -> Switch/2
  Delay/1 -> Sum/2
  Latch/1(Out1) -> Sum/1
  Chirp Signal/1(Out2) -> Multiport Switch/4
  Ramp/1(Out1) -> Multiport Switch/3
  Sum/1 -> Double chirp/1(In1), Double-step/1(Start Time), Chirp Signal/1(Start Time), Ramp/1(Start Time), Step/1(Start Time)
  Maneuver/1 -> Multiport Switch/1
  Step/1(Out) -> Multiport Switch/2
  Amplitude/1 -> Product/3
  Multiport Switch/1 -> Product/2
  Product/1 -> Offset/1
  Product1/1 -> Latch/Trigger, Product/1
  Digital Clock/1 -> Latch/1(In1)
  Switch/1 -> Product1/1
  Constant1/1 -> Switch/3
  Constant/1 -> Switch/1

== system p1_digital_twin_R2023a/Vehicle Chassis Dynamics/Lateral Brush Tire Model/Sgn with deadband ==
  In : Inport
  Dead Zone : DeadZone  LowerValue=-lower_dz  UpperValue=upper_dz  ZeroCross=off
  Sign : Signum  ZeroCross=off
  Out : Outport  VectorParamsAs1DForOutWhenUnconnected=off
  wires:
  In/1 -> Dead Zone/1
  Dead Zone/1 -> Sign/1
  Sign/1 -> Out/1

== system p1_digital_twin_R2023a/Vehicle Chassis Dynamics/WFT Emulation/WFT Byte Packing ==
  In1 : Inport
  Data Type Conversion2 : DataTypeConversion  OutDataTypeStr=int16  SaturateOnIntegerOverflow=off  RndMeth=Floor
  S-Function Builder2 : S-Function  FunctionName=int16ToBytes  SFunctionModules=int16ToBytes_wrapper.c  SFunctionDeploymentMode=off  EnableBusSupport=off  mask(S-Function Builder){}
      mask help: Simulink:masks:SFunctionBuilder_MD
      mask init: same as p1_digital_twin_R2023a/Actuator Dynamics/Steering System Emulation/S-Function Builder1
      settings: CopyFcn=set_param(gcbh,'LinkStatus','none')  OpenFcn=sfunctionwizard(gcbh)
      mask Display:
      | plot(val(:,1),val(:,2))
      | disp(sys)
      | port_label('input',1,'u0')
      | port_label('output',1,'y0')
      | port_label('output',2,'y1')
  WFT Fy unscaling : Gain  Gain=1/0.6103515625
  Out1 : Outport
  Out2 : Outport  Port=2
  wires:
  WFT Fy unscaling/1 -> Data Type Conversion2/1
  Data Type Conversion2/1 -> S-Function Builder2/1
  S-Function Builder2/1 -> Out2/1, Out1/1
  In1/1 -> WFT Fy unscaling/1

== system p1_digital_twin_R2023a/Vehicle Chassis Dynamics/WFT Emulation/WFT Byte Packing1 ==
  In1 : Inport
  Data Type Conversion2 : DataTypeConversion  OutDataTypeStr=int16  SaturateOnIntegerOverflow=off  RndMeth=Floor
  S-Function Builder2 : S-Function  FunctionName=int16ToBytes  SFunctionModules=int16ToBytes_wrapper.c  SFunctionDeploymentMode=off  EnableBusSupport=off  mask(S-Function Builder){}
      mask help: Simulink:masks:SFunctionBuilder_MD
      mask init: same as p1_digital_twin_R2023a/Actuator Dynamics/Steering System Emulation/S-Function Builder1
      settings: CopyFcn=set_param(gcbh,'LinkStatus','none')  OpenFcn=sfunctionwizard(gcbh)
      mask Display:
      | plot(val(:,1),val(:,2))
      | disp(sys)
      | port_label('input',1,'u0')
      | port_label('output',1,'y0')
      | port_label('output',2,'y1')
  WFT Fy unscaling : Gain  Gain=1/0.6103515625
  Out1 : Outport
  Out2 : Outport  Port=2
  wires:
  WFT Fy unscaling/1 -> Data Type Conversion2/1
  Data Type Conversion2/1 -> S-Function Builder2/1
  S-Function Builder2/1 -> Out2/1, Out1/1
  In1/1 -> WFT Fy unscaling/1

== system p1_digital_twin_R2023a/Vehicle Chassis Dynamics/WFT Emulation/WFT Byte Packing10 ==
  In1 : Inport
  Data Type Conversion2 : DataTypeConversion  OutDataTypeStr=int16  SaturateOnIntegerOverflow=off  RndMeth=Floor
  S-Function Builder2 : S-Function  FunctionName=int16ToBytes  SFunctionModules=int16ToBytes_wrapper.c  SFunctionDeploymentMode=off  EnableBusSupport=off  mask(S-Function Builder){}
      mask help: Simulink:masks:SFunctionBuilder_MD
      mask init: same as p1_digital_twin_R2023a/Actuator Dynamics/Steering System Emulation/S-Function Builder1
      settings: CopyFcn=set_param(gcbh,'LinkStatus','none')  OpenFcn=sfunctionwizard(gcbh)
      mask Display:
      | plot(val(:,1),val(:,2))
      | disp(sys)
      | port_label('input',1,'u0')
      | port_label('output',1,'y0')
      | port_label('output',2,'y1')
  WFT Fy unscaling : Gain  Gain=1/0.6103515625
  Out1 : Outport
  Out2 : Outport  Port=2
  wires:
  In1/1 -> WFT Fy unscaling/1
  S-Function Builder2/1 -> Out2/1, Out1/1
  Data Type Conversion2/1 -> S-Function Builder2/1
  WFT Fy unscaling/1 -> Data Type Conversion2/1

== system p1_digital_twin_R2023a/Vehicle Chassis Dynamics/WFT Emulation/WFT Byte Packing11 ==
  In1 : Inport
  Data Type Conversion2 : DataTypeConversion  OutDataTypeStr=int16  SaturateOnIntegerOverflow=off  RndMeth=Floor
  S-Function Builder2 : S-Function  FunctionName=int16ToBytes  SFunctionModules=int16ToBytes_wrapper.c  SFunctionDeploymentMode=off  EnableBusSupport=off  mask(S-Function Builder){}
      mask help: Simulink:masks:SFunctionBuilder_MD
      mask init: same as p1_digital_twin_R2023a/Actuator Dynamics/Steering System Emulation/S-Function Builder1
      settings: CopyFcn=set_param(gcbh,'LinkStatus','none')  OpenFcn=sfunctionwizard(gcbh)
      mask Display:
      | plot(val(:,1),val(:,2))
      | disp(sys)
      | port_label('input',1,'u0')
      | port_label('output',1,'y0')
      | port_label('output',2,'y1')
  WFT Fy unscaling : Gain  Gain=1/0.6103515625
  Out1 : Outport
  Out2 : Outport  Port=2
  wires:
  In1/1 -> WFT Fy unscaling/1
  S-Function Builder2/1 -> Out2/1, Out1/1
  Data Type Conversion2/1 -> S-Function Builder2/1
  WFT Fy unscaling/1 -> Data Type Conversion2/1

== system p1_digital_twin_R2023a/Vehicle Chassis Dynamics/WFT Emulation/WFT Byte Packing12 ==
  In1 : Inport
  Data Type Conversion2 : DataTypeConversion  OutDataTypeStr=int16  SaturateOnIntegerOverflow=off  RndMeth=Floor
  S-Function Builder2 : S-Function  FunctionName=int16ToBytes  SFunctionModules=int16ToBytes_wrapper.c  SFunctionDeploymentMode=off  EnableBusSupport=off  mask(S-Function Builder){}
      mask help: Simulink:masks:SFunctionBuilder_MD
      mask init: same as p1_digital_twin_R2023a/Actuator Dynamics/Steering System Emulation/S-Function Builder1
      settings: CopyFcn=set_param(gcbh,'LinkStatus','none')  OpenFcn=sfunctionwizard(gcbh)
      mask Display:
      | plot(val(:,1),val(:,2))
      | disp(sys)
      | port_label('input',1,'u0')
      | port_label('output',1,'y0')
      | port_label('output',2,'y1')
  WFT Fy unscaling : Gain  Gain=1/0.6103515625
  Out1 : Outport
  Out2 : Outport  Port=2
  wires:
  WFT Fy unscaling/1 -> Data Type Conversion2/1
  Data Type Conversion2/1 -> S-Function Builder2/1
  S-Function Builder2/1 -> Out2/1, Out1/1
  In1/1 -> WFT Fy unscaling/1

== system p1_digital_twin_R2023a/Vehicle Chassis Dynamics/WFT Emulation/WFT Byte Packing13 ==
  In1 : Inport
  Data Type Conversion2 : DataTypeConversion  OutDataTypeStr=int16  SaturateOnIntegerOverflow=off  RndMeth=Floor
  S-Function Builder2 : S-Function  FunctionName=int16ToBytes  SFunctionModules=int16ToBytes_wrapper.c  SFunctionDeploymentMode=off  EnableBusSupport=off  mask(S-Function Builder){}
      mask help: Simulink:masks:SFunctionBuilder_MD
      mask init: same as p1_digital_twin_R2023a/Actuator Dynamics/Steering System Emulation/S-Function Builder1
      settings: CopyFcn=set_param(gcbh,'LinkStatus','none')  OpenFcn=sfunctionwizard(gcbh)
      mask Display:
      | plot(val(:,1),val(:,2))
      | disp(sys)
      | port_label('input',1,'u0')
      | port_label('output',1,'y0')
      | port_label('output',2,'y1')
  WFT Fy unscaling : Gain  Gain=1/0.6103515625
  Out1 : Outport
  Out2 : Outport  Port=2
  wires:
  WFT Fy unscaling/1 -> Data Type Conversion2/1
  Data Type Conversion2/1 -> S-Function Builder2/1
  S-Function Builder2/1 -> Out2/1, Out1/1
  In1/1 -> WFT Fy unscaling/1

== system p1_digital_twin_R2023a/Vehicle Chassis Dynamics/WFT Emulation/WFT Byte Packing14 ==
  In1 : Inport
  Data Type Conversion2 : DataTypeConversion  OutDataTypeStr=int16  SaturateOnIntegerOverflow=off  RndMeth=Floor
  S-Function Builder2 : S-Function  FunctionName=int16ToBytes  SFunctionModules=int16ToBytes_wrapper.c  SFunctionDeploymentMode=off  EnableBusSupport=off  mask(S-Function Builder){}
      mask help: Simulink:masks:SFunctionBuilder_MD
      mask init: same as p1_digital_twin_R2023a/Actuator Dynamics/Steering System Emulation/S-Function Builder1
      settings: CopyFcn=set_param(gcbh,'LinkStatus','none')  OpenFcn=sfunctionwizard(gcbh)
      mask Display:
      | plot(val(:,1),val(:,2))
      | disp(sys)
      | port_label('input',1,'u0')
      | port_label('output',1,'y0')
      | port_label('output',2,'y1')
  WFT Fy unscaling : Gain  Gain=1/0.6103515625
  Out1 : Outport
  Out2 : Outport  Port=2
  wires:
  WFT Fy unscaling/1 -> Data Type Conversion2/1
  Data Type Conversion2/1 -> S-Function Builder2/1
  S-Function Builder2/1 -> Out2/1, Out1/1
  In1/1 -> WFT Fy unscaling/1

== system p1_digital_twin_R2023a/Vehicle Chassis Dynamics/WFT Emulation/WFT Byte Packing15 ==
  In1 : Inport
  Data Type Conversion2 : DataTypeConversion  OutDataTypeStr=int16  SaturateOnIntegerOverflow=off  RndMeth=Floor
  S-Function Builder2 : S-Function  FunctionName=int16ToBytes  SFunctionModules=int16ToBytes_wrapper.c  SFunctionDeploymentMode=off  EnableBusSupport=off  mask(S-Function Builder){}
      mask help: Simulink:masks:SFunctionBuilder_MD
      mask init: same as p1_digital_twin_R2023a/Actuator Dynamics/Steering System Emulation/S-Function Builder1
      settings: CopyFcn=set_param(gcbh,'LinkStatus','none')  OpenFcn=sfunctionwizard(gcbh)
      mask Display:
      | plot(val(:,1),val(:,2))
      | disp(sys)
      | port_label('input',1,'u0')
      | port_label('output',1,'y0')
      | port_label('output',2,'y1')
  WFT Fy unscaling : Gain  Gain=1/0.6103515625
  Out1 : Outport
  Out2 : Outport  Port=2
  wires:
  WFT Fy unscaling/1 -> Data Type Conversion2/1
  Data Type Conversion2/1 -> S-Function Builder2/1
  S-Function Builder2/1 -> Out2/1, Out1/1
  In1/1 -> WFT Fy unscaling/1

== system p1_digital_twin_R2023a/Vehicle Chassis Dynamics/WFT Emulation/WFT Byte Packing16 ==
  In1 : Inport
  Data Type Conversion2 : DataTypeConversion  OutDataTypeStr=int16  SaturateOnIntegerOverflow=off  RndMeth=Floor
  S-Function Builder2 : S-Function  FunctionName=int16ToBytes  SFunctionModules=int16ToBytes_wrapper.c  SFunctionDeploymentMode=off  EnableBusSupport=off  mask(S-Function Builder){}
      mask help: Simulink:masks:SFunctionBuilder_MD
      mask init: same as p1_digital_twin_R2023a/Actuator Dynamics/Steering System Emulation/S-Function Builder1
      settings: CopyFcn=set_param(gcbh,'LinkStatus','none')  OpenFcn=sfunctionwizard(gcbh)
      mask Display:
      | plot(val(:,1),val(:,2))
      | disp(sys)
      | port_label('input',1,'u0')
      | port_label('output',1,'y0')
      | port_label('output',2,'y1')
  WFT Fy unscaling : Gain  Gain=1/0.6103515625
  Out1 : Outport
  Out2 : Outport  Port=2
  wires:
  In1/1 -> WFT Fy unscaling/1
  S-Function Builder2/1 -> Out2/1, Out1/1
  Data Type Conversion2/1 -> S-Function Builder2/1
  WFT Fy unscaling/1 -> Data Type Conversion2/1

== system p1_digital_twin_R2023a/Vehicle Chassis Dynamics/WFT Emulation/WFT Byte Packing17 ==
  In1 : Inport
  Data Type Conversion2 : DataTypeConversion  OutDataTypeStr=int16  SaturateOnIntegerOverflow=off  RndMeth=Floor
  S-Function Builder2 : S-Function  FunctionName=int16ToBytes  SFunctionModules=int16ToBytes_wrapper.c  SFunctionDeploymentMode=off  EnableBusSupport=off  mask(S-Function Builder){}
      mask help: Simulink:masks:SFunctionBuilder_MD
      mask init: same as p1_digital_twin_R2023a/Actuator Dynamics/Steering System Emulation/S-Function Builder1
      settings: CopyFcn=set_param(gcbh,'LinkStatus','none')  OpenFcn=sfunctionwizard(gcbh)
      mask Display:
      | plot(val(:,1),val(:,2))
      | disp(sys)
      | port_label('input',1,'u0')
      | port_label('output',1,'y0')
      | port_label('output',2,'y1')
  WFT Fy unscaling : Gain  Gain=1/0.6103515625
  Out1 : Outport
  Out2 : Outport  Port=2
  wires:
  In1/1 -> WFT Fy unscaling/1
  S-Function Builder2/1 -> Out2/1, Out1/1
  Data Type Conversion2/1 -> S-Function Builder2/1
  WFT Fy unscaling/1 -> Data Type Conversion2/1

== system p1_digital_twin_R2023a/Vehicle Chassis Dynamics/WFT Emulation/WFT Byte Packing18 ==
  In1 : Inport
  Data Type Conversion2 : DataTypeConversion  OutDataTypeStr=int16  SaturateOnIntegerOverflow=off  RndMeth=Floor
  S-Function Builder2 : S-Function  FunctionName=int16ToBytes  SFunctionModules=int16ToBytes_wrapper.c  SFunctionDeploymentMode=off  EnableBusSupport=off  mask(S-Function Builder){}
      mask help: Simulink:masks:SFunctionBuilder_MD
      mask init: same as p1_digital_twin_R2023a/Actuator Dynamics/Steering System Emulation/S-Function Builder1
      settings: CopyFcn=set_param(gcbh,'LinkStatus','none')  OpenFcn=sfunctionwizard(gcbh)
      mask Display:
      | plot(val(:,1),val(:,2))
      | disp(sys)
      | port_label('input',1,'u0')
      | port_label('output',1,'y0')
      | port_label('output',2,'y1')
  WFT Fy unscaling : Gain  Gain=1/0.6103515625
  Out1 : Outport
  Out2 : Outport  Port=2
  wires:
  In1/1 -> WFT Fy unscaling/1
  S-Function Builder2/1 -> Out2/1, Out1/1
  Data Type Conversion2/1 -> S-Function Builder2/1
  WFT Fy unscaling/1 -> Data Type Conversion2/1

== system p1_digital_twin_R2023a/Vehicle Chassis Dynamics/WFT Emulation/WFT Byte Packing19 ==
  In1 : Inport
  Data Type Conversion2 : DataTypeConversion  OutDataTypeStr=int16  SaturateOnIntegerOverflow=off  RndMeth=Floor
  S-Function Builder2 : S-Function  FunctionName=int16ToBytes  SFunctionModules=int16ToBytes_wrapper.c  SFunctionDeploymentMode=off  EnableBusSupport=off  mask(S-Function Builder){}
      mask help: Simulink:masks:SFunctionBuilder_MD
      mask init: same as p1_digital_twin_R2023a/Actuator Dynamics/Steering System Emulation/S-Function Builder1
      settings: CopyFcn=set_param(gcbh,'LinkStatus','none')  OpenFcn=sfunctionwizard(gcbh)
      mask Display:
      | plot(val(:,1),val(:,2))
      | disp(sys)
      | port_label('input',1,'u0')
      | port_label('output',1,'y0')
      | port_label('output',2,'y1')
  WFT Fy unscaling : Gain  Gain=1/0.6103515625
  Out1 : Outport
  Out2 : Outport  Port=2
  wires:
  WFT Fy unscaling/1 -> Data Type Conversion2/1
  Data Type Conversion2/1 -> S-Function Builder2/1
  S-Function Builder2/1 -> Out2/1, Out1/1
  In1/1 -> WFT Fy unscaling/1

== system p1_digital_twin_R2023a/Vehicle Chassis Dynamics/WFT Emulation/WFT Byte Packing2 ==
  In1 : Inport
  Data Type Conversion2 : DataTypeConversion  OutDataTypeStr=int16  SaturateOnIntegerOverflow=off  RndMeth=Floor
  S-Function Builder2 : S-Function  FunctionName=int16ToBytes  SFunctionModules=int16ToBytes_wrapper.c  SFunctionDeploymentMode=off  EnableBusSupport=off  mask(S-Function Builder){}
      mask help: Simulink:masks:SFunctionBuilder_MD
      mask init: same as p1_digital_twin_R2023a/Actuator Dynamics/Steering System Emulation/S-Function Builder1
      settings: CopyFcn=set_param(gcbh,'LinkStatus','none')  OpenFcn=sfunctionwizard(gcbh)
      mask Display:
      | plot(val(:,1),val(:,2))
      | disp(sys)
      | port_label('input',1,'u0')
      | port_label('output',1,'y0')
      | port_label('output',2,'y1')
  WFT Fy unscaling : Gain  Gain=1/0.6103515625
  Out1 : Outport
  Out2 : Outport  Port=2
  wires:
  In1/1 -> WFT Fy unscaling/1
  S-Function Builder2/1 -> Out2/1, Out1/1
  Data Type Conversion2/1 -> S-Function Builder2/1
  WFT Fy unscaling/1 -> Data Type Conversion2/1

== system p1_digital_twin_R2023a/Vehicle Chassis Dynamics/WFT Emulation/WFT Byte Packing3 ==
  In1 : Inport
  Data Type Conversion2 : DataTypeConversion  OutDataTypeStr=int16  SaturateOnIntegerOverflow=off  RndMeth=Floor
  S-Function Builder2 : S-Function  FunctionName=int16ToBytes  SFunctionModules=int16ToBytes_wrapper.c  SFunctionDeploymentMode=off  EnableBusSupport=off  mask(S-Function Builder){}
      mask help: Simulink:masks:SFunctionBuilder_MD
      mask init: same as p1_digital_twin_R2023a/Actuator Dynamics/Steering System Emulation/S-Function Builder1
      settings: CopyFcn=set_param(gcbh,'LinkStatus','none')  OpenFcn=sfunctionwizard(gcbh)
      mask Display:
      | plot(val(:,1),val(:,2))
      | disp(sys)
      | port_label('input',1,'u0')
      | port_label('output',1,'y0')
      | port_label('output',2,'y1')
  WFT Fy unscaling : Gain  Gain=1/0.6103515625
  Out1 : Outport
  Out2 : Outport  Port=2
  wires:
  In1/1 -> WFT Fy unscaling/1
  S-Function Builder2/1 -> Out2/1, Out1/1
  Data Type Conversion2/1 -> S-Function Builder2/1
  WFT Fy unscaling/1 -> Data Type Conversion2/1

== system p1_digital_twin_R2023a/Vehicle Chassis Dynamics/WFT Emulation/WFT Byte Packing4 ==
  In1 : Inport
  Data Type Conversion2 : DataTypeConversion  OutDataTypeStr=int16  SaturateOnIntegerOverflow=off  RndMeth=Floor
  S-Function Builder2 : S-Function  FunctionName=int16ToBytes  SFunctionModules=int16ToBytes_wrapper.c  SFunctionDeploymentMode=off  EnableBusSupport=off  mask(S-Function Builder){}
      mask help: Simulink:masks:SFunctionBuilder_MD
      mask init: same as p1_digital_twin_R2023a/Actuator Dynamics/Steering System Emulation/S-Function Builder1
      settings: CopyFcn=set_param(gcbh,'LinkStatus','none')  OpenFcn=sfunctionwizard(gcbh)
      mask Display:
      | plot(val(:,1),val(:,2))
      | disp(sys)
      | port_label('input',1,'u0')
      | port_label('output',1,'y0')
      | port_label('output',2,'y1')
  WFT Fy unscaling : Gain  Gain=1/0.6103515625
  Out1 : Outport
  Out2 : Outport  Port=2
  wires:
  In1/1 -> WFT Fy unscaling/1
  S-Function Builder2/1 -> Out2/1, Out1/1
  Data Type Conversion2/1 -> S-Function Builder2/1
  WFT Fy unscaling/1 -> Data Type Conversion2/1

== system p1_digital_twin_R2023a/Vehicle Chassis Dynamics/WFT Emulation/WFT Byte Packing5 ==
  In1 : Inport
  Data Type Conversion2 : DataTypeConversion  OutDataTypeStr=int16  SaturateOnIntegerOverflow=off  RndMeth=Floor
  S-Function Builder2 : S-Function  FunctionName=int16ToBytes  SFunctionModules=int16ToBytes_wrapper.c  SFunctionDeploymentMode=off  EnableBusSupport=off  mask(S-Function Builder){}
      mask help: Simulink:masks:SFunctionBuilder_MD
      mask init: same as p1_digital_twin_R2023a/Actuator Dynamics/Steering System Emulation/S-Function Builder1
      settings: CopyFcn=set_param(gcbh,'LinkStatus','none')  OpenFcn=sfunctionwizard(gcbh)
      mask Display:
      | plot(val(:,1),val(:,2))
      | disp(sys)
      | port_label('input',1,'u0')
      | port_label('output',1,'y0')
      | port_label('output',2,'y1')
  WFT Fy unscaling : Gain  Gain=1/0.6103515625
  Out1 : Outport
  Out2 : Outport  Port=2
  wires:
  In1/1 -> WFT Fy unscaling/1
  S-Function Builder2/1 -> Out2/1, Out1/1
  Data Type Conversion2/1 -> S-Function Builder2/1
  WFT Fy unscaling/1 -> Data Type Conversion2/1

== system p1_digital_twin_R2023a/Vehicle Chassis Dynamics/WFT Emulation/WFT Byte Packing6 ==
  In1 : Inport
  Data Type Conversion2 : DataTypeConversion  OutDataTypeStr=int16  SaturateOnIntegerOverflow=off  RndMeth=Floor
  S-Function Builder2 : S-Function  FunctionName=int16ToBytes  SFunctionModules=int16ToBytes_wrapper.c  SFunctionDeploymentMode=off  EnableBusSupport=off  mask(S-Function Builder){}
      mask help: Simulink:masks:SFunctionBuilder_MD
      mask init: same as p1_digital_twin_R2023a/Actuator Dynamics/Steering System Emulation/S-Function Builder1
      settings: CopyFcn=set_param(gcbh,'LinkStatus','none')  OpenFcn=sfunctionwizard(gcbh)
      mask Display:
      | plot(val(:,1),val(:,2))
      | disp(sys)
      | port_label('input',1,'u0')
      | port_label('output',1,'y0')
      | port_label('output',2,'y1')
  WFT Fy unscaling : Gain  Gain=1/0.6103515625
  Out1 : Outport
  Out2 : Outport  Port=2
  wires:
  WFT Fy unscaling/1 -> Data Type Conversion2/1
  Data Type Conversion2/1 -> S-Function Builder2/1
  S-Function Builder2/1 -> Out2/1, Out1/1
  In1/1 -> WFT Fy unscaling/1
